simulink model "e06"  (R2023b)
settings: Solver=VariableStepAuto  StartTime=0.0  StopTime=1000  RelTol=1e-3
values from neighbouring files (symbols this model uses):
  a = 1/33    (= 0.030303030303)    [e00.m]
  b = 1/33000    (= 3.0303030303e-05)    [e00.m]
  c = 0    [e00.m]
  d = 100/33    (= 3.0303030303)    [e00.m]
  f = 1/5    (= 0.2)    [e00.m]
  g = 1/5    (= 0.2)    [e00.m]
  kp = 0.17    [e00.m]
  td = 38    [e00.m]
  ti = 100    [e00.m]
  y_b = 100    [e00.m]
settings Model: Creator=jitbitan  LastModifiedBy=Anirvan Krishna

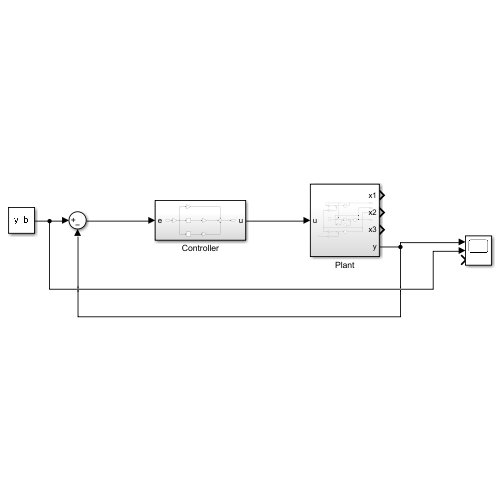
[thumbnail: Simulink's stored preview of the top-level diagram]
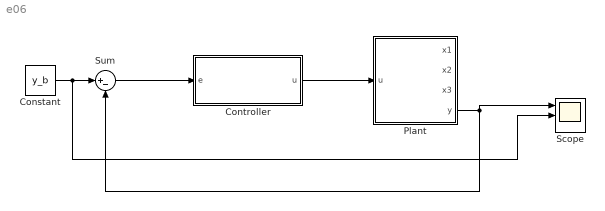
== system e06 ==
  Constant : Constant  Value=y_b
  Controller : Subsystem
  Plant : Subsystem
  Scope : Scope  NumInputPorts=3
  Sum : Sum  Inputs=|+-
  wires:
  Constant/1 -> Scope/2, Sum/1
  Plant/4(y) -> Scope/1, Sum/2
  Controller/1(u) -> Plant/1(u)
  Sum/1 -> Controller/1(e)

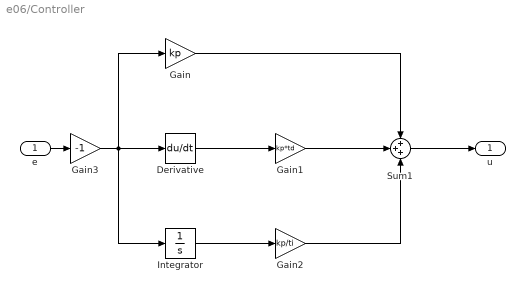
== system e06/Controller ==
  e : Inport
  Derivative : Derivative
  Gain : Gain  Gain=kp
  Gain1 : Gain  Gain=kp*td
  Gain2 : Gain  Gain=kp/ti
  Gain3 : Gain  Gain=-1
  Integrator : Integrator
  Sum1 : Sum  Inputs=+++
  u : Outport
  wires:
  e/1 -> Gain3/1
  Sum1/1 -> u/1
  Gain/1 -> Sum1/1
  Derivative/1 -> Gain1/1
  Gain1/1 -> Sum1/2
  Integrator/1 -> Gain2/1
  Gain2/1 -> Sum1/3
  Gain3/1 -> Derivative/1, Integrator/1, Gain/1

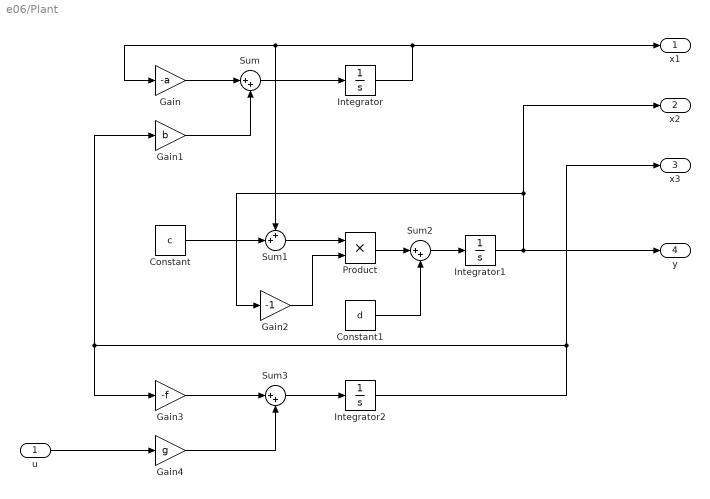
== system e06/Plant ==
  u : Inport
  Constant : Constant  Value=c
  Constant1 : Constant  Value=d
  Gain : Gain  Gain=-a
  Gain1 : Gain  Gain=b
  Gain2 : Gain  Gain=-1
  Gain3 : Gain  Gain=-f
  Gain4 : Gain  Gain=g
  Integrator : Integrator
  Integrator1 : Integrator
  Integrator2 : Integrator
  Product : Product
  Sum : Sum  Inputs=|++
  Sum1 : Sum  Inputs=++|
  Sum2 : Sum  Inputs=|++
  Sum3 : Sum  Inputs=|++
  x1 : Outport
  x2 : Outport  Port=2
  x3 : Outport  Port=3
  y : Outport  Port=4
  wires:
  Constant1/1 -> Sum2/2
  Gain4/1 -> Sum3/2
  Integrator1/1 -> y/1, x2/1, Gain2/1
  Sum3/1 -> Integrator2/1
  Integrator2/1 -> x3/1, Gain1/1, Gain3/1
  Integrator/1 -> x1/1, Gain/1, Sum1/1
  Gain/1 -> Sum/1
  Sum2/1 -> Integrator1/1
  Product/1 -> Sum2/1
  Constant/1 -> Sum1/2
  Sum/1 -> Integrator/1
  Gain1/1 -> Sum/2
  Gain2/1 -> Product/2
  Sum1/1 -> Product/1
  Gain3/1 -> Sum3/1
  u/1 -> Gain4/1
